simulink model "SMC_AC_Quadcopter_Simulation_ver3"  (R2013b)
settings: Solver=FixedStepDiscrete  StartTime=0  StopTime=10  FixedStep=0.025  MaxStep=0.06  RelTol=1e-3
model workspace (MAT data in the model file):
  Sig = Simulink.Signal
  Sig.DataType = 'auto'
  Sig.Dimensions = -1
  Sig.DimensionsMode = 'auto'
  Sig.Complexity = 'auto'
  Sig.SampleTime = -1
  Sig.SamplingMode = 'auto'
values from neighbouring files (symbols this model uses):
  IC = block.DialogPrm(2).Data    [quadcopterDynamicsSFunction.m]
undefined symbols (not defined in the file or in its folder): quadModel, sigbuilder_block
Description:
  | This is a configurable quadcopter simulation.
  | This Simulink model demonstates attitude control.
  | 
  | Additional quadcopter modeling and simulation materials available at:
  | github.com/dch33/Quad-Sim
  | 
  | Copyright (C) 2014 D. Hartman, K. Landis, S. Moreno, J. Kim, M. Mehrer
  | 
  | License:
  |     This program is free software: you can redistribute it and/or modify
  |     it under the terms of the GNU LESSER GENERAL PUBLIC LICENSE as published by
  |     the Free Software Foundation, either version 3 of the License, or
  |     (at your option) any later version.
  | 
  |     This program is distributed in the hope that it will be useful,
  |     but WITHOUT ANY WARRANTY; without even the implied warranty of
  |     MERCHANTABILITY or FITNESS FOR A PARTICULAR PURPOSE.  See the
  |     GNU General Public License for more details.
  | 
  |     You should have received a copy of the GNU LESSER GENERAL PUBLIC LICENSE
  |     along with this program.  If not, see <http://www.gnu.org/licenses/>.
settings Model: ModifiedComment=SwiftWind -- Sat Jun 04 20:07:49 2016 -- Version 1.8  Creator=David Hartman  LastModifiedBy=SwiftWind
settings Model: ModifiedHistory=|
  | SwiftWind -- Sat Jun 04 20:07:49 2016 -- Version 1.8
  | 
  | 
  | SwiftWind -- Sat Jun 04 19:15:30 2016 -- Version 1.7
  | 
  | 
  | Sliding Mode Control of Quadrotor's Attitude
  | 
  | SwiftWind -- Sat Jun 04 16:15:53 2016 -- Version 1.6
  | 
  | davidhartman -- Fri Jun 06 23:19:51 2014 -- Version 1.5
  | 
  | 
  | davidhartman -- Fri Jun 06 22:53:10 2014 -- Version 1.3
settings SolverCC: AutoInsertRateTranBlk=on
settings DataIOCC: LimitDataPoints=off  SignalLogging=off
settings OptimizationCC: DefaultParameterBehavior=Inlined  SimCompilerOptimization=off
settings DebuggingCC: FrameProcessingCompatibilityMsg=error  UniqueDataStoreMsg=warning  StateNameClashWarn=warning  StrictBusMsg=WarnOnBusTreatedAsVector
settings RTWCC: RTWCompilerOptimization=off
settings GRTTargetCC: TargetLangStandard=C89/C90 (ANSI)  CodeReplacementLibrary=None  CPPClassGenCompliant=on
settings ConfigComp: CovMetricSettings=dw  CovHtmlReporting=on  CovSaveCumulativeToWorkspaceVar=on  CovSaveSingleToWorkspaceVar=on  CovModelRefEnable=Off  CovExternalEMLEnable=off

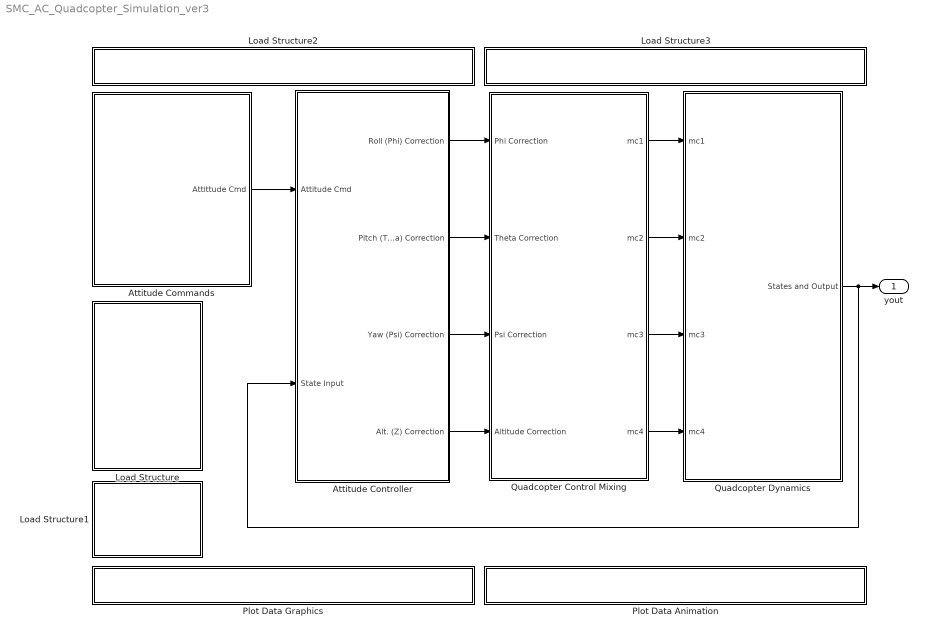
== system SMC_AC_Quadcopter_Simulation_ver3 ==
  Attitude Commands : Subsystem
  Attitude Controller : Subsystem
  Load Structure : Subsystem
      settings: OpenFcn=|
      | uiopen('load')
      | if (exist('IC')==1 && exist('quadModel')==1)
      | set_param(bdroot, 'SimulationCommand', 'update')
      | end
      mask Display: fprintf('LOAD:\nQuadcopter\nModel Or\nInitial\nConditions');
  Load Structure1 : Subsystem
      settings: OpenFcn=|
      | if (exist('IC')==1 && exist('quadModel')==1 && exist('yout') && exist('tout'))
      | saveSimResults()
      | else
      | msgbox('No Data To Save!')
      | end
      mask Display: fprintf('SAVE:\nSimulation\nResults');
  Load Structure2 : Subsystem
      settings: OpenFcn=|
      | if exist('GUI_Modeling') == 2,
      | run('GUI_Modeling')
      | 
      | else
      | 
      | msgbox('The desired GUI must be first added to MATLABs path.')
      | 
      | end
      mask Display: fprintf('OPEN GUI: Build New \n Model');
  Load Structure3 : Subsystem
      settings: OpenFcn=|
      | if exist('GUI_IC') == 2,
      | run('GUI_IC')
      | 
      | else
      | 
      | msgbox('The desired GUI must be first added to MATLABs path.')
      | 
      | end
      mask Display: fprintf('OPEN GUI: Create Initial \n Conditions');
  Plot Data Animation : Subsystem
      settings: OpenFcn=|
      | if exist('QuadAnim4') == 2,
      |     if exist('yout')
      | 	run('QuadAnim4');
      |     else
      |     msgbox('Simulation must be run before data can be plotted.');
      |     end
      | else                                                                          msgbox('The desired GUI must be first added to MATLABs path.')
      | end
      mask Display: fprintf('OPEN GUI: Flight Animation')
  Plot Data Graphics : Subsystem
      settings: OpenFcn=|
      | if exist('yout')
      | yout = evalin('base', 'yout');
      | tout = evalin('base', 'tout');
      | quadPlots(yout, tout)
      | else
      | msgbox('Simulation must be run before data can be plotted.')
      | end
      mask Display: fprintf('OPEN PLOT: State Data')
  Quadcopter Control Mixing : Subsystem
      mask Display:
      | modelLoaded = evalin('base','exist(''quadModel'',''var'')');
      | if (modelLoaded==1)
      |     if (evalin('base','quadModel.plusConfig'))
      |     fprintf([' \n' ' \n'  'Configuration "+"']);
      |     else if (~evalin('base','quadModel.plusConfig'))
      |         fprintf([' \n' ' \n' 'Configuration "X"']);
      |         end
      |     end
      | else
      |     fprintf([' \n' ' \n'  'Model Not Loaded']);
      | end
  Quadcopter Dynamics : Subsystem
  yout : Outport
  wires:
  Quadcopter Dynamics/1(States and Output) -> yout/1, Attitude Controller/2(State Input)
  Quadcopter Control Mixing/1(mc1) -> Quadcopter Dynamics/1(mc1)
  Quadcopter Control Mixing/2(mc2) -> Quadcopter Dynamics/2(mc2)
  Quadcopter Control Mixing/3(mc3) -> Quadcopter Dynamics/3(mc3)
  Quadcopter Control Mixing/4(mc4) -> Quadcopter Dynamics/4(mc4)
  Attitude Controller/1(Roll (Phi) Correction) -> Quadcopter Control Mixing/1(Phi Correction)
  Attitude Controller/2(Pitch (Theta) Correction) -> Quadcopter Control Mixing/2(Theta Correction)
  Attitude Controller/3(Yaw (Psi) Correction) -> Quadcopter Control Mixing/3(Psi Correction)
  Attitude Controller/4(Alt. (Z) Correction) -> Quadcopter Control Mixing/4(Altitude Correction)
  Attitude Commands/1(Attittude Cmd) -> Attitude Controller/1(Attitude Cmd)

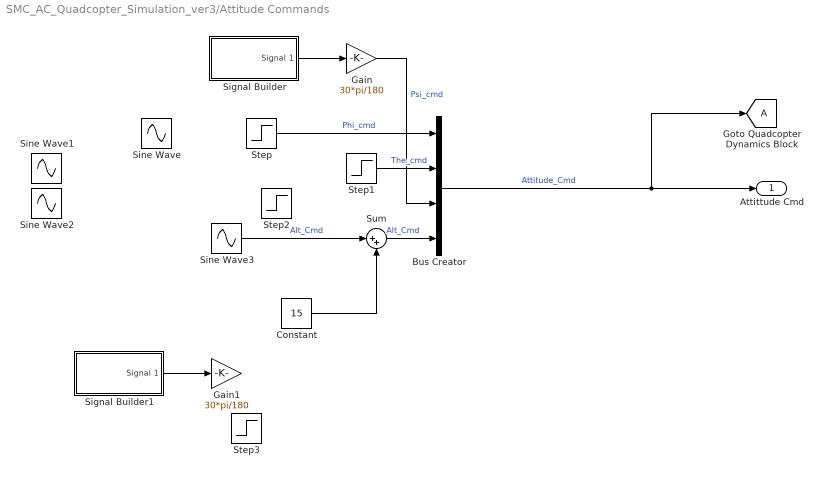
== system SMC_AC_Quadcopter_Simulation_ver3/Attitude Commands ==
  Bus Creator : BusCreator
  Constant : Constant  Value=15
  Gain : Gain  Gain=30*pi/180
  Gain1 : Gain  Gain=30*pi/180
  Signal Builder : Subsystem  Tag=STV Subsys  LoadFcn=sigbuilder_block('load');  StartFcn=sigbuilder_block('start');  StopFcn=sigbuilder_block('stop');  ClipboardFcn=sigbuilder_block('clipboard');  mask(Sigbuilder block){}
      mask help: Simulink:masks:SigbuilderBlock_MD
      mask init:
      | if ~strcmp(get_param(bdroot(gcbh),'SimulationStatus'),'stopped') tuvar = sigbuilder_block('maskInit'); end
      settings: CopyFcn=sigbuilder_block('copy');  DeleteFcn=sigbuilder_block('delete');  ModelCloseFcn=sigbuilder_block('modelClose');  PreSaveFcn=sigbuilder_block('preSave');  PauseFcn=sigbuilder_block('pause');  ContinueFcn=sigbuilder_block('continue');  NameChangeFcn=sigbuilder_block('namechange');  OpenFcn=sigbuilder_block('open',[437.25 199.5 550.5 399.75 ]);  CloseFcn=sigbuilder_block('close');
      mask Display: plot(0, 0, 100, 100,[2, 2, 32, 32, 2], [68, 8, 8, 68, 68],[32, 2], [38, 38], [32, 19, 2],[53, 60, 44], [32, 17, 17, 2],[16, 16, 31, 31]);txt = getActiveGroup(gcbh);text(2, 100, txt,'verticalAlignment', 'top');
  Signal Builder1 : Subsystem  Tag=STV Subsys  LoadFcn=sigbuilder_block('load');  StartFcn=sigbuilder_block('start');  StopFcn=sigbuilder_block('stop');  ClipboardFcn=sigbuilder_block('clipboard');  mask(Sigbuilder block){}
      mask help: Simulink:masks:SigbuilderBlock_MD
      mask init:
      | if ~strcmp(get_param(bdroot(gcbh),'SimulationStatus'),'stopped') tuvar = sigbuilder_block('maskInit'); end
      settings: CopyFcn=sigbuilder_block('copy');  DeleteFcn=sigbuilder_block('delete');  ModelCloseFcn=sigbuilder_block('modelClose');  PreSaveFcn=sigbuilder_block('preSave');  PauseFcn=sigbuilder_block('pause');  ContinueFcn=sigbuilder_block('continue');  NameChangeFcn=sigbuilder_block('namechange');  OpenFcn=sigbuilder_block('open',[437.25 199.5 550.5 399.75 ]);  CloseFcn=sigbuilder_block('close');
      mask Display: plot(0, 0, 100, 100,[2, 2, 32, 32, 2], [68, 8, 8, 68, 68],[32, 2], [38, 38], [32, 19, 2],[53, 60, 44], [32, 17, 17, 2],[16, 16, 31, 31]);txt = getActiveGroup(gcbh);text(2, 100, txt,'verticalAlignment', 'top');
  Sine Wave : Sin  SampleTime=0
  Sine Wave1 : Sin  Amplitude=0  Frequency=.1  SampleTime=0
  Sine Wave2 : Sin  Amplitude=0  SampleTime=0
  Sine Wave3 : Sin  Amplitude=0  Frequency=.5  SampleTime=0
  Step : Step  Time=0  After=0*pi/180  SampleTime=0
  Step1 : Step  Time=0  After=0*pi/180  SampleTime=0
  Step2 : Step  Time=7  After=0*pi/180  SampleTime=0
  Step3 : Step  Time=5  Before=100  After=100  SampleTime=0
  Sum : Sum  Inputs=|++
  Attittude Cmd : Outport
  tag scope: A=global
  wires:
  Bus Creator/1 -> Attittude Cmd/1, [A]  "Attitude_Cmd"
  Constant/1 -> Sum/2
  Sine Wave3/1 -> Sum/1  "Alt_Cmd"
  Sum/1 -> Bus Creator/4  "Alt_Cmd"
  Signal Builder/1(Signal 1) -> Gain/1
  Signal Builder1/1(Signal 1) -> Gain1/1
  Step/1 -> Bus Creator/1  "Phi_cmd"
  Step1/1 -> Bus Creator/2  "The_cmd"
  Gain/1 -> Bus Creator/3  "Psi_cmd"

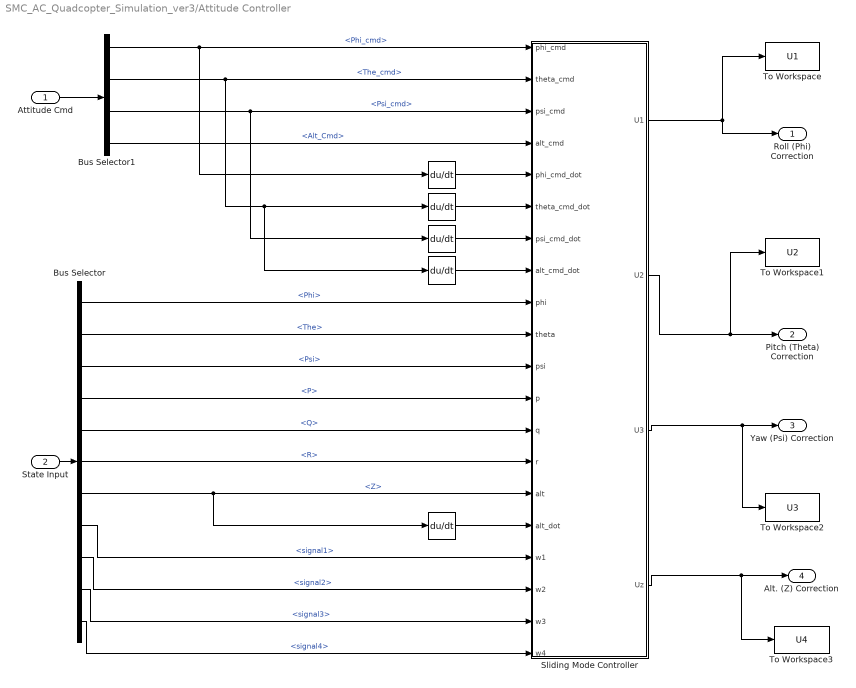
== system SMC_AC_Quadcopter_Simulation_ver3/Attitude Controller ==
  Attitude Cmd : Inport
  State Input : Inport  Port=2
  " " : Derivative
  " " : Derivative
  "    " : Derivative
  "      " : Derivative
  "        " : Derivative
  Bus Selector : BusSelector  OutputSignals=Phi,The,Psi,P,Q,R,Z,mc and RPM.signal1,mc and RPM.signal2,mc and RPM.signal3,mc and RPM.signal4
  Bus Selector1 : BusSelector  OutputSignals=Phi_cmd,The_cmd,Psi_cmd,Alt_Cmd
  Sliding Mode Controller : MATLAB Function  TreatAsAtomicUnit=on
  To Workspace : ToWorkspace  VariableName=U1  SampleTime=-1  SaveFormat=Timeseries
  To Workspace1 : ToWorkspace  VariableName=U2  SampleTime=-1  SaveFormat=Timeseries
  To Workspace2 : ToWorkspace  VariableName=U3  SampleTime=-1  SaveFormat=Timeseries
  To Workspace3 : ToWorkspace  VariableName=U4  SampleTime=-1  SaveFormat=Timeseries
  Roll (Phi) Correction : Outport
  Pitch (Theta) Correction : Outport  Port=2
  Yaw (Psi) Correction : Outport  Port=3
  Alt. (Z) Correction : Outport  Port=4
  wires:
  Bus Selector/6 -> Sliding Mode Controller/14(r)  "<R>"
  Bus Selector/5 -> Sliding Mode Controller/13(q)  "<Q>"
  Bus Selector/2 -> Sliding Mode Controller/10(theta)  "<The>"
  Bus Selector/3 -> Sliding Mode Controller/11(psi)  "<Psi>"
  State Input/1 -> Bus Selector/1
  Bus Selector/8 -> Sliding Mode Controller/17(w1)  "<signal1>"
  Bus Selector/9 -> Sliding Mode Controller/18(w2)  "<signal2>"
  Bus Selector/10 -> Sliding Mode Controller/19(w3)  "<signal3>"
  Bus Selector/11 -> Sliding Mode Controller/20(w4)  "<signal4>"
  Bus Selector/1 -> Sliding Mode Controller/9(phi)  "<Phi>"
  Bus Selector/7 -> Sliding Mode Controller/15(alt), "        "/1  "<Z>"
  Bus Selector/4 -> Sliding Mode Controller/12(p)  "<P>"
  Attitude Cmd/1 -> Bus Selector1/1
  Bus Selector1/1 -> Sliding Mode Controller/1(phi_cmd), " "/1  "<Phi_cmd>"
  Bus Selector1/2 -> " "/1, "      "/1, Sliding Mode Controller/2(theta_cmd)  "<The_cmd>"
  Bus Selector1/3 -> "    "/1, Sliding Mode Controller/3(psi_cmd)  "<Psi_cmd>"
  Bus Selector1/4 -> Sliding Mode Controller/4(alt_cmd)  "<Alt_Cmd>"
  " "/1 -> Sliding Mode Controller/5(phi_cmd_dot)
  " "/1 -> Sliding Mode Controller/6(theta_cmd_dot)
  "    "/1 -> Sliding Mode Controller/7(psi_cmd_dot)
  "      "/1 -> Sliding Mode Controller/8(alt_cmd_dot)
  Sliding Mode Controller/4(Uz) -> To Workspace3/1, Alt. (Z) Correction/1
  Sliding Mode Controller/1(U1) -> Roll (Phi) Correction/1, To Workspace/1
  Sliding Mode Controller/2(U2) -> To Workspace1/1, Pitch (Theta) Correction/1
  Sliding Mode Controller/3(U3) -> Yaw (Psi) Correction/1, To Workspace2/1
  "        "/1 -> Sliding Mode Controller/16(alt_dot)

== system SMC_AC_Quadcopter_Simulation_ver3/Load Structure ==

== system SMC_AC_Quadcopter_Simulation_ver3/Load Structure1 ==

== system SMC_AC_Quadcopter_Simulation_ver3/Load Structure2 ==

== system SMC_AC_Quadcopter_Simulation_ver3/Load Structure3 ==

== system SMC_AC_Quadcopter_Simulation_ver3/Plot Data Animation ==

== system SMC_AC_Quadcopter_Simulation_ver3/Plot Data Graphics ==

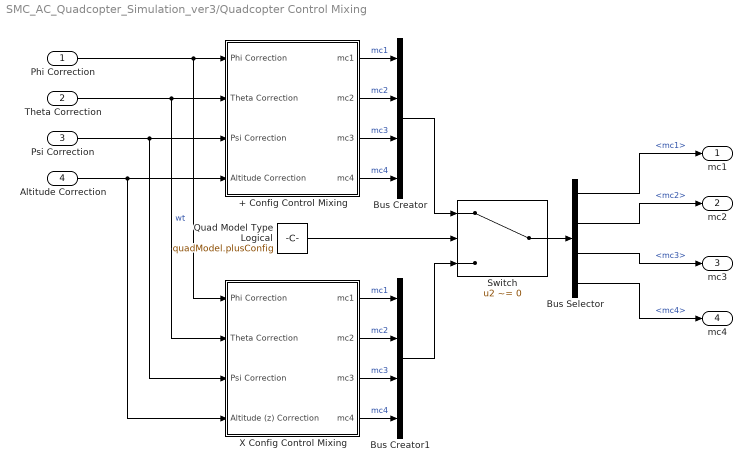
== system SMC_AC_Quadcopter_Simulation_ver3/Quadcopter Control Mixing ==
  Phi Correction : Inport
  Theta Correction : Inport  Port=2
  Psi Correction : Inport  Port=3
  Altitude Correction : Inport  Port=4
  + Config Control Mixing : Subsystem
  Bus Creator : BusCreator
  Bus Creator1 : BusCreator
  Bus Selector : BusSelector  OutputSignals=mc1,mc2,mc3,mc4
  Quad Model Type Logical : Constant  Value=quadModel.plusConfig
  Switch : Switch  Criteria=u2 ~= 0
  X Config Control Mixing : Subsystem
  mc1 : Outport
  mc2 : Outport  Port=2
  mc3 : Outport  Port=3
  mc4 : Outport  Port=4
  wires:
  Switch/1 -> Bus Selector/1
  Quad Model Type Logical/1 -> Switch/2
  Bus Selector/4 -> mc4/1  "<mc4>"
  Bus Selector/3 -> mc3/1  "<mc3>"
  Bus Selector/2 -> mc2/1  "<mc2>"
  Bus Selector/1 -> mc1/1  "<mc1>"
  Bus Creator1/1 -> Switch/3
  X Config Control Mixing/4(mc4) -> Bus Creator1/4  "mc4"
  X Config Control Mixing/3(mc3) -> Bus Creator1/3  "mc3"
  X Config Control Mixing/2(mc2) -> Bus Creator1/2  "mc2"
  X Config Control Mixing/1(mc1) -> Bus Creator1/1  "mc1"
  Bus Creator/1 -> Switch/1
  + Config Control Mixing/4(mc4) -> Bus Creator/4  "mc4"
  + Config Control Mixing/3(mc3) -> Bus Creator/3  "mc3"
  + Config Control Mixing/2(mc2) -> Bus Creator/2  "mc2"
  + Config Control Mixing/1(mc1) -> Bus Creator/1  "mc1"
  Altitude Correction/1 -> + Config Control Mixing/4(Altitude Correction), X Config Control Mixing/4(Altitude (z) Correction)
  Psi Correction/1 -> + Config Control Mixing/3(Psi Correction), X Config Control Mixing/3(Psi Correction)
  Theta Correction/1 -> + Config Control Mixing/2(Theta Correction), X Config Control Mixing/2(Theta Correction)  "wt"
  Phi Correction/1 -> + Config Control Mixing/1(Phi Correction), X Config Control Mixing/1(Phi Correction)

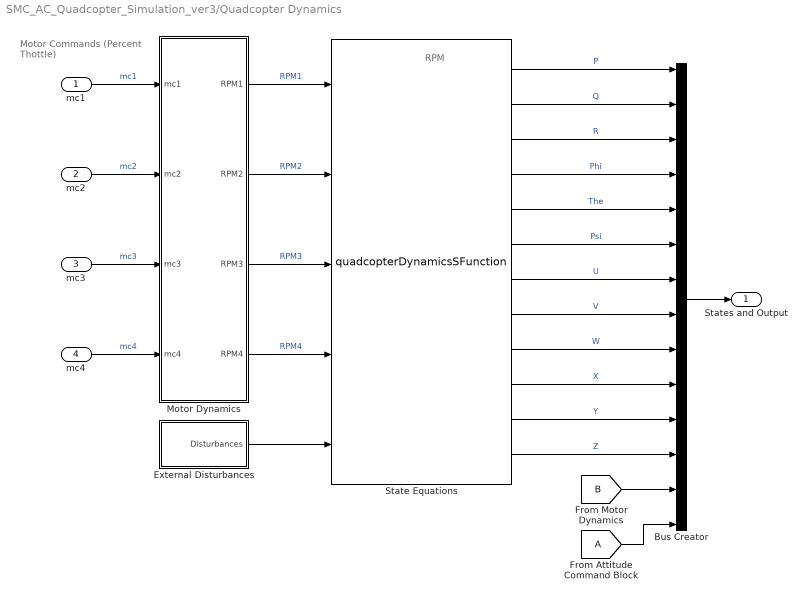
== system SMC_AC_Quadcopter_Simulation_ver3/Quadcopter Dynamics ==
  note: Motor Commands
      | (Percent Thottle)
  note: RPM
  mc1 : Inport
  mc2 : Inport  Port=2
  mc3 : Inport  Port=3
  mc4 : Inport  Port=4
  Bus Creator : BusCreator  Inputs='P','Q','R','Phi','The','Psi','U','V','W','X','Y','Z','mc and RPM','Attitude_Cmd'
  External Disturbances : Subsystem
  Motor Dynamics : Subsystem
  State Equations : M-S-Function  FunctionName=quadcopterDynamicsSFunction  Parameters=quadModel, IC
      mask Display:
      | port_label('input', 1, 'RPM1')
      | port_label('input', 2, 'RPM2')
      | port_label('input', 3, 'RPM3')
      | port_label('input', 4, 'RPM4')
      | port_label('input', 5, 'Disturbances')
      | port_label('output', 1, 'P')
      | port_label('output', 2, 'Q')
      | port_label('output', 3, 'R')
      | port_label('output', 4, 'Phi')
      | port_label('output', 5, 'The')
      | port_label('output', 6, 'Psi')
      | port_label('output', 7, 'U')
      | port_label('output', 8, 'V')
      | port_label('output', 9, 'W')
      | port_label('output', 10, 'X')
      | port_label('output', 11, 'Y')
      | port_label('output', 12, 'Z')
  States and Output : Outport
  wires:
  [B] -> Bus Creator/13
  [A] -> Bus Creator/14
  External Disturbances/1("Disturbances ") -> State Equations/5
  mc2/1 -> Motor Dynamics/2(mc2)  "mc2"
  mc3/1 -> Motor Dynamics/3(mc3)  "mc3"
  mc4/1 -> Motor Dynamics/4(mc4)  "mc4"
  mc1/1 -> Motor Dynamics/1(mc1)  "mc1"
  Motor Dynamics/4(RPM4) -> State Equations/4  "RPM4"
  Motor Dynamics/3(RPM3) -> State Equations/3  "RPM3"
  Motor Dynamics/2(RPM2) -> State Equations/2  "RPM2"
  Motor Dynamics/1(RPM1) -> State Equations/1  "RPM1"
  Bus Creator/1 -> States and Output/1
  State Equations/12 -> Bus Creator/12  "Z"
  State Equations/11 -> Bus Creator/11  "Y"
  State Equations/10 -> Bus Creator/10  "X"
  State Equations/9 -> Bus Creator/9  "W"
  State Equations/8 -> Bus Creator/8  "V"
  State Equations/7 -> Bus Creator/7  "U"
  State Equations/6 -> Bus Creator/6  "Psi"
  State Equations/5 -> Bus Creator/5  "The"
  State Equations/4 -> Bus Creator/4  "Phi"
  State Equations/3 -> Bus Creator/3  "R"
  State Equations/2 -> Bus Creator/2  "Q"
  State Equations/1 -> Bus Creator/1  "P"

== system SMC_AC_Quadcopter_Simulation_ver3/Attitude Commands/Signal Builder ==
  Demux : Demux  Tag=STV Demux  Outputs=1
  FromWs : FromWorkspace  Tag=STV FromWs  VariableName=tuvar  SampleTime=0
      SigBuilderData=|
      | common.afterFinalStr = 'Extrapolate'
      | common.sampleTime = 0
      | dataSet.timeRange = [0 10]
      | dataSet.name = 'Group 1'
      | sbobj.Groups.Name = 'Group 1'
      | sbobj.Groups.Signals.Name = 'Signal 1'
      | sbobj.Groups.Signals.XData = [0 4 4 6 6 8 8 10]
      | sbobj.Groups.Signals.YData = [0 0 1 1 -1 -1 0 0]
  Signal 1 : Outport  Tag=STV Outport
  wires:
  Demux/1 -> Signal 1/1
  FromWs/1 -> Demux/1

== system SMC_AC_Quadcopter_Simulation_ver3/Attitude Commands/Signal Builder1 ==
  Demux : Demux  Tag=STV Demux  Outputs=1
  FromWs : FromWorkspace  Tag=STV FromWs  VariableName=tuvar  SampleTime=0
      SigBuilderData=|
      | common.afterFinalStr = 'Extrapolate'
      | common.sampleTime = 0
      | dataSet.timeRange = [0 10]
      | dataSet.name = 'Group 1'
      | sbobj.Groups.Name = 'Group 1'
      | sbobj.Groups.Signals.Name = 'Signal 1'
      | sbobj.Groups.Signals.XData = [0 4 4 6 6 8 8 10]
      | sbobj.Groups.Signals.YData = [0 0 1 1 -1 -1 0 0]
  Signal 1 : Outport  Tag=STV Outport
  wires:
  FromWs/1 -> Demux/1
  Demux/1 -> Signal 1/1

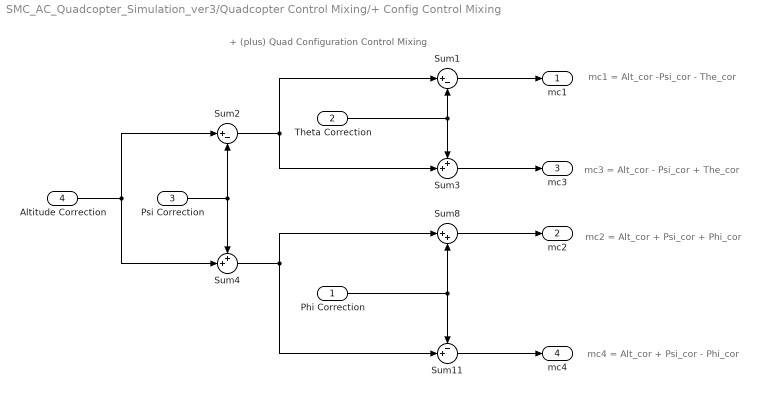
== system SMC_AC_Quadcopter_Simulation_ver3/Quadcopter Control Mixing/+ Config Control Mixing ==
  note: mc1 = Alt_cor -Psi_cor - The_cor
  note: mc3 = Alt_cor - Psi_cor + The_cor
  note: mc4 = Alt_cor + Psi_cor - Phi_cor
  note: + (plus) Quad Configuration Control Mixing
  note: mc2 = Alt_cor + Psi_cor + Phi_cor
  Phi Correction : Inport
  Theta Correction : Inport  Port=2
  Psi Correction : Inport  Port=3
  Altitude Correction : Inport  Port=4
  Sum1 : Sum  Inputs=|+-
  Sum11 : Sum  Inputs=-+|
  Sum2 : Sum  Inputs=|+-
  Sum3 : Sum  Inputs=++|
  Sum4 : Sum  Inputs=++|
  Sum8 : Sum  Inputs=|++
  mc1 : Outport
  mc2 : Outport  Port=2
  mc3 : Outport  Port=3
  mc4 : Outport  Port=4
  wires:
  Sum11/1 -> mc4/1
  Sum8/1 -> mc2/1
  Sum3/1 -> mc3/1
  Sum1/1 -> mc1/1
  Phi Correction/1 -> Sum11/1, Sum8/2
  Sum4/1 -> Sum8/1, Sum11/2
  Psi Correction/1 -> Sum2/2, Sum4/1
  Sum2/1 -> Sum1/1, Sum3/2
  Altitude Correction/1 -> Sum4/2, Sum2/1
  Theta Correction/1 -> Sum3/1, Sum1/2

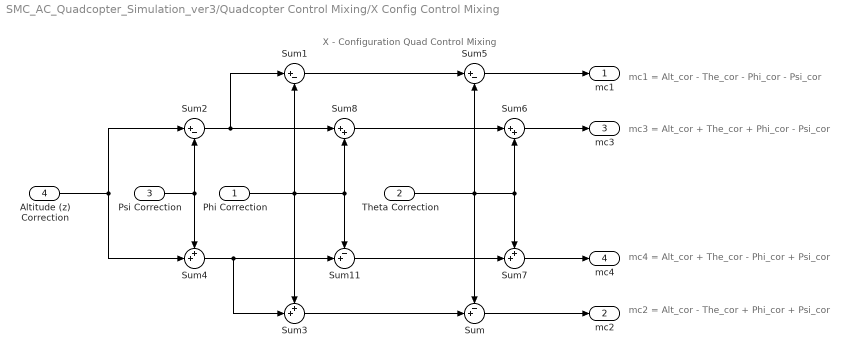
== system SMC_AC_Quadcopter_Simulation_ver3/Quadcopter Control Mixing/X Config Control Mixing ==
  note: mc4 = Alt_cor + The_cor - Phi_cor + Psi_cor
  note: mc2 = Alt_cor - The_cor + Phi_cor + Psi_cor
  note: mc3 = Alt_cor + The_cor + Phi_cor - Psi_cor
  note: X - Configuration Quad Control Mixing
  note: mc1 = Alt_cor - The_cor - Phi_cor - Psi_cor
  Phi Correction : Inport
  Theta Correction : Inport  Port=2
  Psi Correction : Inport  Port=3
  Altitude (z) Correction : Inport  Port=4
  Sum : Sum  Inputs=-+|
  Sum1 : Sum  Inputs=|+-
  Sum11 : Sum  Inputs=-+|
  Sum2 : Sum  Inputs=|+-
  Sum3 : Sum  Inputs=++|
  Sum4 : Sum  Inputs=++|
  Sum5 : Sum  Inputs=|+-
  Sum6 : Sum  Inputs=|++
  Sum7 : Sum  Inputs=++|
  Sum8 : Sum  Inputs=|++
  mc1 : Outport
  mc2 : Outport  Port=2
  mc3 : Outport  Port=3
  mc4 : Outport  Port=4
  wires:
  Sum/1 -> mc2/1
  Altitude (z) Correction/1 -> Sum4/2, Sum2/1
  Sum7/1 -> mc4/1
  Sum6/1 -> mc3/1
  Sum5/1 -> mc1/1
  Sum11/1 -> Sum7/2
  Sum8/1 -> Sum6/1
  Sum1/1 -> Sum5/1
  Theta Correction/1 -> Sum/1, Sum5/2, Sum6/2, Sum7/1
  Sum3/1 -> Sum/2
  Sum4/1 -> Sum11/2, Sum3/2
  Phi Correction/1 -> Sum11/1, Sum8/2, Sum1/2, Sum3/1
  Psi Correction/1 -> Sum2/2, Sum4/1
  Sum2/1 -> Sum1/1, Sum8/1

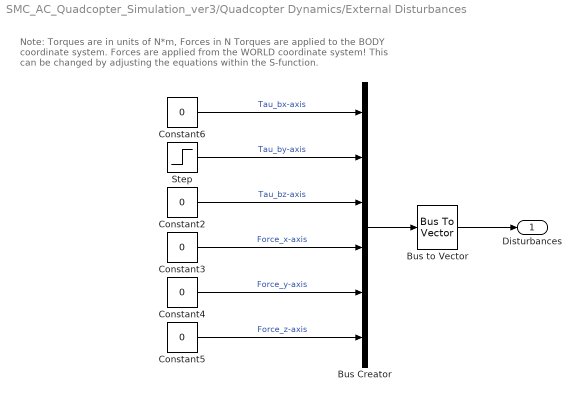
== system SMC_AC_Quadcopter_Simulation_ver3/Quadcopter Dynamics/External Disturbances ==
  note: Note: Torques are in units of N*m, Forces in N
      | Torques are applied to the BODY coordinate system.
      | Forces are applied from the WORLD coordinate system!
      | This can be changed by adjusting the equations within the S-function.
  Bus Creator : BusCreator  Inputs=6
  Bus to Vector : BusToVector
  Constant{2..6} (5 alike) : Constant  Value=0
  Step : Step  Time=0  After=0  SampleTime=0
  "Disturbances " : Outport
  wires:
  Constant5/1 -> Bus Creator/6  "Force_z-axis"
  Constant4/1 -> Bus Creator/5  "Force_y-axis"
  Constant3/1 -> Bus Creator/4  "Force_x-axis"
  Constant2/1 -> Bus Creator/3  "Tau_bz-axis"
  Step/1 -> Bus Creator/2  "Tau_by-axis"
  Constant6/1 -> Bus Creator/1  "Tau_bx-axis"
  Bus Creator/1 -> Bus to Vector/1
  Bus to Vector/1 -> "Disturbances "/1

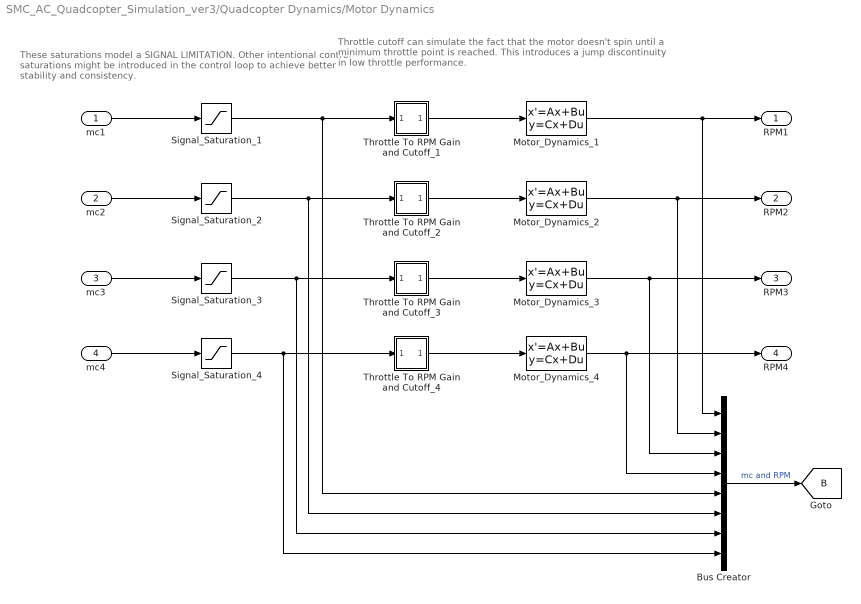
== system SMC_AC_Quadcopter_Simulation_ver3/Quadcopter Dynamics/Motor Dynamics ==
  note: These saturations model a SIGNAL LIMITATION.
      | Other intentional control saturations might be introduced in the
      | control loop to achieve better stability and consistency.
  note: Throttle cutoff can simulate the fact that the motor doesn't
      | spin until a minimum throttle point is reached. This introduces
      | a jump discontinuity in low throttle performance.
  mc1 : Inport
  mc2 : Inport  Port=2
  mc3 : Inport  Port=3
  mc4 : Inport  Port=4
  Bus Creator : BusCreator  Inputs=8
  Motor_Dynamics_1 : StateSpace  A=-1/quadModel.T  C=1/quadModel.T  D=0  X0=IC.w1*quadModel.T
  Motor_Dynamics_2 : StateSpace  A=-1/quadModel.T  C=1/quadModel.T  D=0  X0=IC.w2*quadModel.T
  Motor_Dynamics_3 : StateSpace  A=-1/quadModel.T  C=1/quadModel.T  D=0  X0=IC.w3*quadModel.T
  Motor_Dynamics_4 : StateSpace  A=-1/quadModel.T  C=1/quadModel.T  D=0  X0=IC.w4*quadModel.T
  Signal_Saturation_{1..4} (4 alike) : Saturate  UpperLimit=100  LowerLimit=0
  Throttle To RPM Gain and Cutoff_1 : Subsystem
  Throttle To RPM Gain and Cutoff_2 : Subsystem
  Throttle To RPM Gain and Cutoff_3 : Subsystem
  Throttle To RPM Gain and Cutoff_4 : Subsystem
  RPM1 : Outport
  RPM2 : Outport  Port=2
  RPM3 : Outport  Port=3
  RPM4 : Outport  Port=4
  tag scope: B=global
  wires:
  Bus Creator/1 -> [B]  "mc and RPM"
  Motor_Dynamics_4/1 -> RPM4/1, Bus Creator/4
  Motor_Dynamics_3/1 -> RPM3/1, Bus Creator/3
  Motor_Dynamics_2/1 -> RPM2/1, Bus Creator/2
  Motor_Dynamics_1/1 -> RPM1/1, Bus Creator/1
  Throttle To RPM Gain and Cutoff_4/1(Out5) -> Motor_Dynamics_4/1
  Throttle To RPM Gain and Cutoff_3/1(Out5) -> Motor_Dynamics_3/1
  Throttle To RPM Gain and Cutoff_2/1(Out5) -> Motor_Dynamics_2/1
  Throttle To RPM Gain and Cutoff_1/1(Out5) -> Motor_Dynamics_1/1
  Signal_Saturation_4/1 -> Throttle To RPM Gain and Cutoff_4/1(In5), Bus Creator/8
  Signal_Saturation_3/1 -> Throttle To RPM Gain and Cutoff_3/1(In5), Bus Creator/7
  Signal_Saturation_2/1 -> Throttle To RPM Gain and Cutoff_2/1(In5), Bus Creator/6
  Signal_Saturation_1/1 -> Throttle To RPM Gain and Cutoff_1/1(In5), Bus Creator/5
  mc3/1 -> Signal_Saturation_3/1
  mc2/1 -> Signal_Saturation_2/1
  mc4/1 -> Signal_Saturation_4/1
  mc1/1 -> Signal_Saturation_1/1

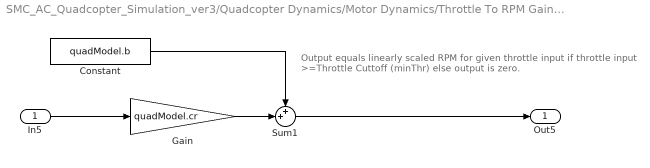
== system SMC_AC_Quadcopter_Simulation_ver3/Quadcopter Dynamics/Motor Dynamics/Throttle To RPM Gain and Cutoff_1 ==
  note: Output equals linearly scaled RPM
      | for given throttle input if throttle input >=Throttle Cuttoff (minThr)
      | else output is zero.
  In5 : Inport
  Constant : Constant  Value=quadModel.b
  Gain : Gain  Gain=quadModel.cr
  Sum1 : Sum  Inputs=++|
  Out5 : Outport
  wires:
  Constant/1 -> Sum1/1
  Gain/1 -> Sum1/2
  In5/1 -> Gain/1
  Sum1/1 -> Out5/1

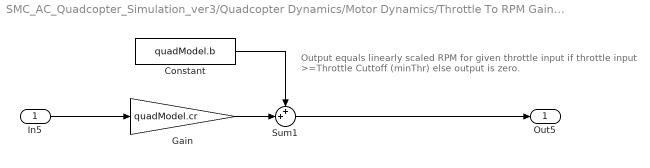
== system SMC_AC_Quadcopter_Simulation_ver3/Quadcopter Dynamics/Motor Dynamics/Throttle To RPM Gain and Cutoff_2 ==
  note: Output equals linearly scaled RPM
      | for given throttle input if throttle input >=Throttle Cuttoff (minThr)
      | else output is zero.
  In5 : Inport
  Constant : Constant  Value=quadModel.b
  Gain : Gain  Gain=quadModel.cr
  Sum1 : Sum  Inputs=++|
  Out5 : Outport
  wires:
  Constant/1 -> Sum1/1
  Gain/1 -> Sum1/2
  In5/1 -> Gain/1
  Sum1/1 -> Out5/1

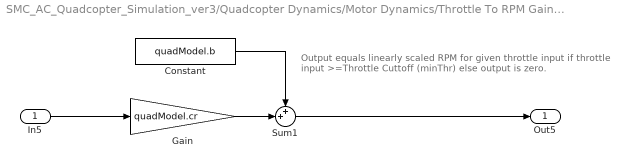
== system SMC_AC_Quadcopter_Simulation_ver3/Quadcopter Dynamics/Motor Dynamics/Throttle To RPM Gain and Cutoff_3 ==
  note: Output equals linearly scaled RPM
      | for given throttle input if throttle input >=Throttle Cuttoff (minThr)
      | else output is zero.
  In5 : Inport
  Constant : Constant  Value=quadModel.b
  Gain : Gain  Gain=quadModel.cr
  Sum1 : Sum  Inputs=++|
  Out5 : Outport
  wires:
  Constant/1 -> Sum1/1
  Gain/1 -> Sum1/2
  In5/1 -> Gain/1
  Sum1/1 -> Out5/1

== system SMC_AC_Quadcopter_Simulation_ver3/Quadcopter Dynamics/Motor Dynamics/Throttle To RPM Gain and Cutoff_4 ==
  note: Output equals linearly scaled RPM
      | for given throttle input if throttle input >=Throttle Cuttoff (minThr)
      | else output is zero.
  In5 : Inport
  Constant : Constant  Value=quadModel.b
  Gain : Gain  Gain=quadModel.cr
  Sum1 : Sum  Inputs=++|
  Out5 : Outport
  wires:
  Constant/1 -> Sum1/1
  Gain/1 -> Sum1/2
  In5/1 -> Gain/1
  Sum1/1 -> Out5/1

== matlab function SMC_AC_Quadcopter_Simulation_ver3/Attitude Controller/Sliding Mode Controller ==
  data: phi_cmd input; theta_cmd input; psi_cmd input; alt_cmd input; phi_cmd_dot input; theta_cmd_dot input; psi_cmd_dot input; alt_cmd_dot input; phi input; theta input; psi input; U1 output; p input; q input; r input; alt input; alt_dot input; w1 input; w2 input; w3 input; w4 input; U2 output; U3 output; Uz output
%% Sliding Mode for Attitude Control of Quadrotor
% z : New State for Tracking Control (Command - Feedback)
function [U1,U2,U3, Uz]  = SMC_Attitude(phi_cmd, theta_cmd, psi_cmd, alt_cmd, phi_cmd_dot, theta_cmd_dot, psi_cmd_dot, alt_cmd_dot, phi, theta, psi, p, q, r, alt, alt_dot,w1, w2, w3, w4)
%% SMC Initial Setup
% Retrieve Parameter from Model
% Ix = Model.Jx;
% Iy = Model.Jy;
% Iz = Model.Jz;
Jr = 3.441e-04; % Propeller Inertia Using 2/3*MR^2 [kg*m^2]
% l = Model.arms_L; % Quadrotor CoG to Motor Length

Ix = [0.0132610000000000];
Iy = [0.0132610000000000];
Iz = [0.0253620000000000];
l = 0.25;
m = 1.05;

a1 = (Iy-Iz)/Ix;
a2 = Jr/Ix;
a3 = (Iz-Ix)/Iy;
a4 = Jr/Iy;
a5 = (Ix-Iy)/Iz;


b1 = l/Ix;
b2 = l/Iy;
b3 = 1/Iz;

OMG_r = (w1 + w3 - w2 - w4) * 2*pi/60; 
% Motors Ang. Vel. Expressing Gyroscopic Forces [rad/s]

%% SMC Control Gains
% % Roll Controller Gains
% alpha1 = 2;
% % K1 = [30 15];
% K1 = [16 8];
% % Pitch Controller Gains
% % is same as Roll Control due to Symmetry
% alpha2 = alpha1;
% K2 = K1;
% 
% % Yaw Controller Gains
% alpha3 = 2;
% K3 = [30 15];
% 
% % Altitude Controller Gains
% alpha_z = 5;
% Kz = [20 3];
% SMC Control Gains
% Roll Controller Gains
alpha1 = 5;
% K1 = [25 50];
% K1 = [16 8];
K1 = [30 60];
% Pitch Controller Gains
% is same as Roll Control due to Symmetry
alpha2 = 10;
K2 = [30 60];

% Yaw Controller Gains
alpha3 = 5;
K3 = [100 50];

% Altitude Controller Gains
alpha_z = 5;
Kz = [20 3];
%% Sliding Surface
% Sliding Surface for Tracking Control 
% for Roll
z1 = phi_cmd - phi;
% z1 = -z1;
S1 = p - phi_cmd_dot - alpha1*z1; 

% for Theta
z2 = theta_cmd - theta;
% z2 = -z2;
S2 = q - theta_cmd_dot - alpha2*z2;

% for Psi
z3 = psi_cmd - psi;
% z3 = -z3;
S3 = r - psi_cmd_dot - alpha3*z3;

% for Z 
zz = alt_cmd - alt;
Sz = alt_dot - alt_cmd_dot - alpha_z*zz;

%% Sliding Controller
% a2 = 0; a4 =0;
% Boudallah Thesis Sliding by Backstepping Approach
% U1 = 1/b1*(-a1*q*r - a2*q*OMG_r - alpha1^2*z1 - K1(1)*sat(S1) - K1(2)*S1);
% 
% U2 = 1/b2*(a3*p*r - a4*p*OMG_r - alpha2^2*z2 - K2(1)*sat(S2) - K2(2)*S2);
% 
% U3 = 1/b3*(-a5*p*q - alpha3^2*z3 - K3(1)*sat(S3) - K3(2)*S3);

% Bouadi Paper Sliding Control by Backstepping Approach
U1 = 1/b1*(-a1*q*r + a2*OMG_r*q - K1(1)*sat(S1) - K1(2)*S1 + alpha1*(phi_cmd_dot - p));
U2 = 1/b2*(-a3*p*r - a4*p*OMG_r +alpha2*(theta_cmd_dot - q) -K2(1)*sat(S2) - K2(2)*S2);
U3 = 1/b3*(-a5*p*q - K3(1)*sat(S3) - K3(2)*S3 + alpha3*(psi_cmd_dot-r));
Uz = m/(cos(phi)*cos(theta))*(-Kz(1)*sat(Sz) - Kz(2)*Sz + alpha_z*(alt_cmd_dot - alt_dot) + 9.81);
